simulink model "DataCollector"  (R2024b)
settings: Solver=FixedStepAuto  StartTime=0.0  StopTime=2  FixedStep=0.001  RelTol=1e-3  EnableMultiTasking=on
libraries: stm32f4xxblockslib x3, simulink x1, dspstat3 x1
settings Model: STM32="{\"DigitalPortRead\":[{\"ID\":\"test:4\"},{\"ID\":\"DataCollector:4\"}],\"AnalogInput\":[{\"ID\":\"test:47\"},{\"ID\":\"DataCollector:47\"}],\"DigitalPortWrite\":[{\"ID\":\"test:64\"},{\"ID\":\"DataCollector:64\"}]}"  Creator=FREED  LastModifiedBy=sitanan
settings OptimizationCC: DefaultParameterBehavior=Inlined  EnhancedBackFolding=on  PassReuseOutputArgsAs=Individual arguments  ZeroExternalMemoryAtStartup=off  ZeroInternalMemoryAtStartup=off  MaxStackSize=512  OptimizeBlockOrder=speed  DifferentSizesBufferReuse=on  OptimizationCustomize=off  EfficientTunableParamExpr=on
settings DebuggingCC: ParameterTunabilityLossMsg=error
settings HardwareCC: ProdBitPerPointer=32  ProdBitPerSizeT=32  ProdBitPerPtrDiffT=32  ProdLargestAtomicInteger=Long  ProdLargestAtomicFloat=Double  ProdWordSize=32  ProdLongLongMode=on  ProdHWDeviceType=ARM Compatible->ARM Cortex-M
settings SFSimCC: MATLABDynamicMemAlloc=off
settings RTWCC: Description=Embedded Coder  SystemTargetFile=ert.tlc  HardwareBoard=STM32G4xx Based  TemplateMakefile=ert_default_tmf  Toolchain=GNU Tools for ARM Embedded Processors
settings CodeAppCC: ForceParamTrailComments=on  IgnoreCustomStorageClasses=off  OperatorAnnotations=on  SimulinkDataObjDesc=on  SFDataObjDesc=on  InsertBlockDesc=on
settings ERTTargetCC: TargetLangStandard=C99 (ISO)  CodeReplacementLibrary=ARM Cortex-M  ExtModeTransport=3  ExtModeStaticAlloc=on  ExtModeStaticAllocSize=2048  ExtModeMexFile=ext_xcp  ExtModeIntrfLevel=Level2 - Open

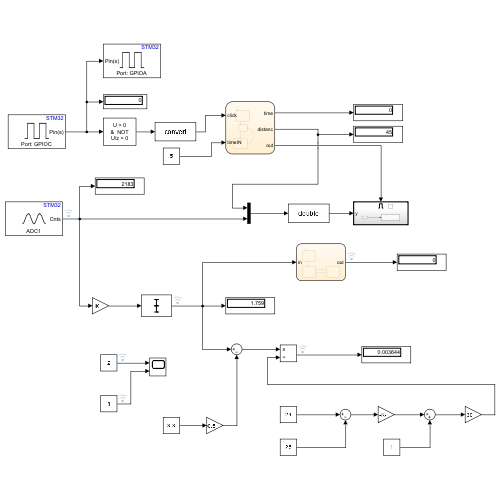
[thumbnail: Simulink's stored preview of the top-level diagram]
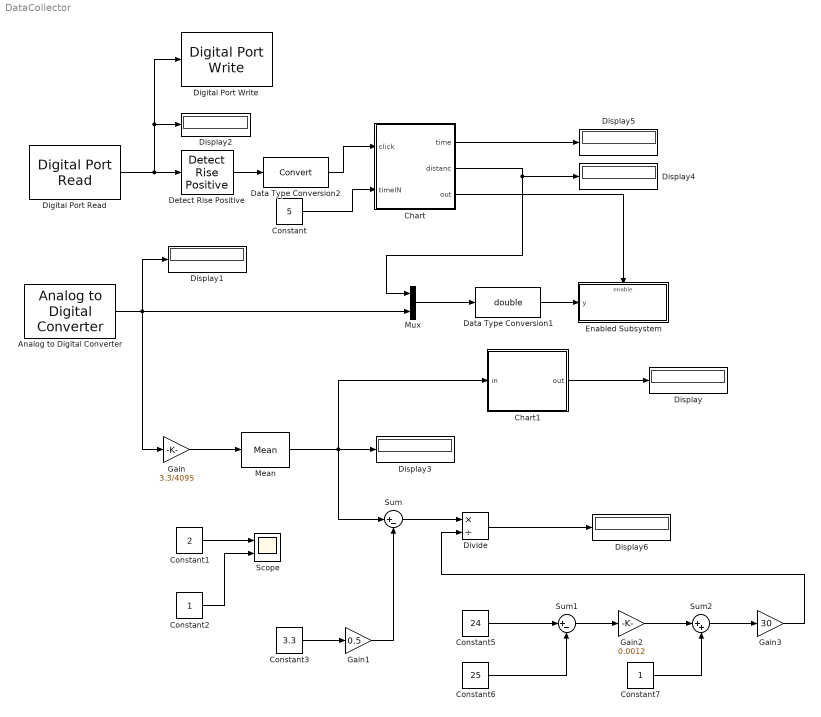
== system DataCollector ==
  Analog to Digital Converter : stm32f4xxblockslib/Analog to Digital Converter  ADCModule=ADC1  ConversionGroup=Regular  TriggerMode=Trigger and read  NumberOfConversions=1  EnableBufferConv=off  BufferLength=1  OutputStatus=off  SampleTime=-1  EnableSimPort=off  hoistedMaskSrc=ECSoC/ECSimCodegen/Analog to Digital Converter
  Chart : Stateflow chart  TreatAsAtomicUnit=on
      settings: PortSchema="{\"entries\":[{\"content\":{\"sides\":[{\"content\":{\"connectorIds\":[\"In1\",\"In2\"]},\"type\":\"ConnectorPlacement.EquallySpacedRectSide\",\"uuid\":\"23737671-6c77-48d5-a6cc-1bdb914c70fb\"},{\"content\":{\"connectorIds\":[\"Out2\",\"Out3\",\"Out1\"],\"side\":\"RIGHT\"},\"type\":\"ConnectorPlacement.EquallySpacedRectSide\",\"uuid\":\"c4f4d2da-48a9-4dbb-99b2-32e79874ad96\"},{\"content\":{\"side\":\"TOP\"},\"type\":\"ConnectorPlacement.EquallySpacedRectSide\",\"uuid\":\"8928c8a6-3a88-4b7e-be4f-b0785bd80b20\"}]},\"type\":\"ConnectorPlacement.EquallySpacedConnector\",\"uuid\":\"35861c40-ff18-4b9a-8c75-1e7eff7ef78b\"}],\"packageUris\":[\"http://schema.mathworks.com/mf0/Connector/R2020b\"],\"version\":\"1.0\"}"
  Chart1 : Stateflow chart  TreatAsAtomicUnit=on
  Constant : Constant  Value=5
  Constant1 : Constant  Value=2
  Constant2 : Constant
  Constant3 : Constant  Value=3.3
  Constant5 : Constant  Value=24
  Constant6 : Constant  Value=25
  Constant7 : Constant
  Data Type Conversion1 : DataTypeConversion  OutDataTypeStr=double  SaturateOnIntegerOverflow=off  RndMeth=Floor
  Data Type Conversion2 : DataTypeConversion  SaturateOnIntegerOverflow=off  RndMeth=Floor
  Detect Rise Positive : simulink/Logic and Bit Operations/Detect Rise Positive  vinit=0  OutDataTypeStr=boolean
  Digital Port Read : stm32f4xxblockslib/Digital Port Read  PortName=GPIOC  PinNumber=[13]  ReadOperation=on  IOAsArray=on  SampleTime=-1  EnableSimPort=off  hoistedMaskSrc=ECSoC/ECSimCodegen/Digital Port Read
      settings: LibrarySourceBlock=stm32g4xxblockslib/Digital Port Read
  Digital Port Write : stm32f4xxblockslib/Digital Port Write  PortName=GPIOA  PinNumber=[5]  ReadOperation=off  IOAsArray=on  EnableSimPort=off  hoistedMaskSrc=ECSoC/ECSimCodegen/Digital Port Write
      settings: LibrarySourceBlock=stm32g4xxblockslib/Digital Port Write
  Display{,1..6} (7 alike) : Display
  Divide : Product  Inputs=*/
  Enabled Subsystem : Subsystem  TreatAsAtomicUnit=on
  Gain : Gain  Gain=3.3/4095
  Gain1 : Gain  Gain=0.5
  Gain2 : Gain  Gain=0.0012
  Gain3 : Gain  Gain=30
  Mean : dspstat3/Mean  run=off  InputProcessing=Columns as channels (frame based)  reset_popup=None  directionMode=Each column  dimension=1  roiEnable=off  roiType=Rectangles  roiPortion=Entire ROI  roiOutput=Individual statistics for each ROI  roiFlag=off  roundingMode=Floor  overflowMode=off  outputDataTypeStr=Inherit: Same as accumulator  outputMin=[]  outputMax=[]  outputLastDataTypeStr=Inherit: Same as accumulator
  Mux : Mux  Inputs=2
  Scope : Scope  NumInputPorts=2
  Sum : Sum  Inputs=|+-
  Sum1 : Sum  Inputs=|+-
  Sum2 : Sum  Inputs=|++
  wires:
  Digital Port Read/1 -> Digital Port Write/1, Display2/1, Detect Rise Positive/1
  Analog to Digital Converter/1 -> Display1/1, Mux/2, Gain/1
  Gain/1 -> Mean/1
  Constant/1 -> Chart/2(timeIN)
  Chart/2(time) -> Display5/1
  Detect Rise Positive/1 -> Data Type Conversion2/1
  Chart/1(out) -> Enabled Subsystem/Enable
  Data Type Conversion2/1 -> Chart/1(click)
  Chart/3(distanc) -> Mux/1, Display4/1
  Mux/1 -> Data Type Conversion1/1
  Data Type Conversion1/1 -> Enabled Subsystem/1(y)
  Mean/1 -> Sum/1, Chart1/1(in), Display3/1
  Chart1/1(out) -> Display/1
  Constant1/1 -> Scope/1
  Constant2/1 -> Scope/2
  Constant3/1 -> Gain1/1
  Gain1/1 -> Sum/2
  Sum/1 -> Divide/1
  Constant5/1 -> Sum1/1
  Constant6/1 -> Sum1/2
  Sum1/1 -> Gain2/1
  Gain2/1 -> Sum2/1
  Constant7/1 -> Sum2/2
  Sum2/1 -> Gain3/1
  Gain3/1 -> Divide/2
  Divide/1 -> Display6/1

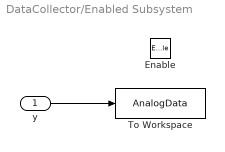
== system DataCollector/Enabled Subsystem ==
  y : Inport
  Enable : EnablePort
  To Workspace : ToWorkspace  VariableName=AnalogData  SampleTime=-1
      settings: Save2DSignal=2-D array (concatenate along first dimension)
  wires:
  y/1 -> To Workspace/1

== stateflow chart DataCollector/Chart1 ==
  state start
    out = 0;
  state low
    entry:
    out = 0;
  state high
    entry:
    out = 3.3;
  (default) -> start
  start -> low : [in <= 1]
  low -> high : [in > 2]
  high -> low : [in < 1.5]
  data: in input; out output

== stateflow chart DataCollector/Chart ==
  state setup
    entry:
    time=0;
    out=0;
    distanc=45;
  state start
    entry:
    time=0;
    out=0;
  state setup1
    entry:
    out=1;
    during:
    time=time+0.01;
    exit:
    distanc=distanc-3
  (default) -> setup
  setup -> start
  setup1 -> start : [time>=timeIN-0.01]
  start -> setup1 : [click == 1]
  data: click input; out output; time output; distanc output; timeIN input
